simulink model "Hell_ix_System_Architecture"  (R2022b)
settings: Solver=VariableStepAuto  StartTime=0.0  StopTime=10.0  RelTol=1e-3
(part 2 of 2)

== system Hell_ix_System_Architecture/Trials/Test 1: In-Line Obstacle Race ==
  Bus Element In4 : Inport  PortName=End1_hellix
  Bus Element In3 : Inport  Port=2  PortName=End1_droning
  Bus Element In2 : Inport  Port=3  PortName=Start
  Bus Element In1 : Inport  Port=4  PortName=obs
  Bus Element Out1 : Outport  PortName=Points1_hellix
  Bus Element Out2 : Outport  Port=2  PortName=Points1_droning

== system Hell_ix_System_Architecture/Trials/Test 2: Semicircle Obstacle Race ==
  Bus Element In4 : Inport  PortName=End2_hellix
  Bus Element In3 : Inport  Port=2  PortName=End2_droning
  Bus Element In2 : Inport  Port=3  PortName=Start
  Bus Element In1 : Inport  Port=4  PortName=obs
  Bus Element Out1 : Outport  PortName=Points2_hellix
  Bus Element Out2 : Outport  Port=2  PortName=Points2_droning

== system Hell_ix_System_Architecture/Trials/Test 3: Freestyle Test ==
  Bus Element In1 : Inport  PortName=Start
  Bus Element In2 : Inport  Port=2  PortName=End
  Bus Element Out1 : Outport  PortName=Points3_hellix
  Bus Element Out2 : Outport  Port=2  PortName=Points3_droning

== system Hell_ix_System_Architecture/Trials/Winner Determination ==
  Bus Element In2 : Inport  PortName=Points1_droning
  Bus Element In1 : Inport  Port=2  PortName=Points1_hellix
  Bus Element In3 : Inport  Port=3  PortName=Points2_hellix
  Bus Element In4 : Inport  Port=4  PortName=Points2_droning
  Bus Element In6 : Inport  Port=5  PortName=Points3_droning
  Bus Element In5 : Inport  Port=6  PortName=Points3_hellix
  Bus Element Out1 : Outport  PortName=Winner

== system Hell_ix_System_Architecture/Environment/Materials/Chronometer ==
  Bus Element In1 : Inport  PortName=Start
  Bus Element Out1 : Outport  PortName=End

== system Hell_ix_System_Architecture/Environment/Materials/Horn ==
  Bus Element Out1 : Outport  PortName=Start

== system Hell_ix_System_Architecture/Environment/Materials/Obstacles ==
  Bus Element Out1 : Outport  PortName=obs

== system Hell_ix_System_Architecture/Environment/Materials/Recording Cameras ==
  Bus Element In2 : Inport  PortName=End
  Bus Element In1 : Inport  Port=2  PortName=Start

== system Hell_ix_System_Architecture/Environment/People/Audience ==

== system Hell_ix_System_Architecture/Environment/People/Droning Team Members ==
  Bus Element In1 : Inport  PortName=Start2
  Control Manager Droning : Subsystem
      settings: PortSchema="{\"entries\":[{\"content\":{\"headerSize\":26,\"margin\":15,\"minimumSpacing\":25,\"sides\":[{\"content\":{\"connectorIds\":[\"In1\"]},\"type\":\"ConnectorPlacement.EquallySpacedRectSide\",\"uuid\":\"e97e1fd1-9f1b-43cc-bf15-a23fe97b9f57\"},{\"content\":{\"connectorIds\":[\"Out1\"],\"side\":\"RIGHT\"},\"type\":\"ConnectorPlacement.EquallySpacedRectSide\",\"uuid\":\"b384b9c5-fcee-4054-b020-18cc4d409726\"},{\"content\":{\"connectorIds\":[],\"side\":\"TOP\"},\"type\":\"ConnectorPlacement.EquallySpacedRectSide\",\"uuid\":\"0ff74274-cc13-4bc9-ab97-befa0144ddb0\"},{\"content\":{\"connectorIds\":[],\"side\":\"BOTTOM\"},\"type\":\"ConnectorPlacement.EquallySpacedRectSide\",\"uuid\":\"4b238d12-a85d-41d6-ac28-0fdf4a244d85\"}]},\"type\":\"ConnectorPlacement.EquallySpacedConnector\",\"uuid\":\"32a64cae-dc0e-47e5-be72-f6041fa7e3a1\"}],\"packageUris\":[\"http://schema.mathworks.com/mf0/Connector/R2020b\"],\"version\":\"1.0\"}"
  Rest of the Droning Team : Subsystem
      settings: PortSchema="{\"entries\":[{\"content\":{\"headerSize\":26,\"margin\":15,\"minimumSpacing\":25,\"sides\":[{\"content\":{\"connectorIds\":[]},\"type\":\"ConnectorPlacement.EquallySpacedRectSide\",\"uuid\":\"e97e1fd1-9f1b-43cc-bf15-a23fe97b9f57\"},{\"content\":{\"connectorIds\":[],\"side\":\"RIGHT\"},\"type\":\"ConnectorPlacement.EquallySpacedRectSide\",\"uuid\":\"b384b9c5-fcee-4054-b020-18cc4d409726\"},{\"content\":{\"connectorIds\":[],\"side\":\"TOP\"},\"type\":\"ConnectorPlacement.EquallySpacedRectSide\",\"uuid\":\"0ff74274-cc13-4bc9-ab97-befa0144ddb0\"}]},\"type\":\"ConnectorPlacement.EquallySpacedConnector\",\"uuid\":\"32a64cae-dc0e-47e5-be72-f6041fa7e3a1\"}],\"packageUris\":[\"http://schema.mathworks.com/mf0/Connector/R2020b\"],\"version\":\"1.0\"}"
  Bus Element Out1 : Outport  PortName=exec_prog2
  wires:
  Bus Element In1/1 -> Control Manager Droning/1(Start2)
  Control Manager Droning/1(exec_prog2) -> Bus Element Out1/1

== system Hell_ix_System_Architecture/Environment/People/Hell-ix Team Members ==
  Bus Element In1 : Inport  PortName=Start
  Control Manager Hell-ix : Subsystem
      settings: PortSchema="{\"entries\":[{\"content\":{\"headerSize\":26,\"margin\":15,\"minimumSpacing\":25,\"sides\":[{\"content\":{\"connectorIds\":[]},\"type\":\"ConnectorPlacement.EquallySpacedRectSide\",\"uuid\":\"e97e1fd1-9f1b-43cc-bf15-a23fe97b9f57\"},{\"content\":{\"connectorIds\":[\"Out1\"],\"side\":\"RIGHT\"},\"type\":\"ConnectorPlacement.EquallySpacedRectSide\",\"uuid\":\"b384b9c5-fcee-4054-b020-18cc4d409726\"},{\"content\":{\"connectorIds\":[\"Out2\"],\"side\":\"TOP\"},\"type\":\"ConnectorPlacement.EquallySpacedRectSide\",\"uuid\":\"0ff74274-cc13-4bc9-ab97-befa0144ddb0\"},{\"content\":{\"connectorIds\":[\"In1\"],\"side\":\"BOTTOM\"},\"type\":\"ConnectorPlacement.EquallySpacedRectSide\",\"uuid\":\"4b238d12-a85d-41d6-ac28-0fdf4a244d85\"}]},\"type\":\"ConnectorPlacement.EquallySpacedConnector\",\"uuid\":\"32a64cae-dc0e-47e5-be72-f6041fa7e3a1\"}],\"packageUris\":[\"http://schema.mathworks.com/mf0/Connector/R2020b\"],\"version\":\"1.0\"}"
  Rest of the Hell-ix Team : Subsystem
      settings: PortSchema="{\"entries\":[{\"content\":{\"headerSize\":26,\"margin\":15,\"minimumSpacing\":25,\"sides\":[{\"content\":{\"connectorIds\":[]},\"type\":\"ConnectorPlacement.EquallySpacedRectSide\",\"uuid\":\"e97e1fd1-9f1b-43cc-bf15-a23fe97b9f57\"},{\"content\":{\"connectorIds\":[],\"side\":\"RIGHT\"},\"type\":\"ConnectorPlacement.EquallySpacedRectSide\",\"uuid\":\"b384b9c5-fcee-4054-b020-18cc4d409726\"},{\"content\":{\"connectorIds\":[],\"side\":\"TOP\"},\"type\":\"ConnectorPlacement.EquallySpacedRectSide\",\"uuid\":\"0ff74274-cc13-4bc9-ab97-befa0144ddb0\"}]},\"type\":\"ConnectorPlacement.EquallySpacedConnector\",\"uuid\":\"32a64cae-dc0e-47e5-be72-f6041fa7e3a1\"}],\"packageUris\":[\"http://schema.mathworks.com/mf0/Connector/R2020b\"],\"version\":\"1.0\"}"
  Bus Element Out1 : Outport  PortName=exec_prog
  Bus Element Out2 : Outport  Port=2  PortName=config
  wires:
  Control Manager Hell-ix/2(exec_prog) -> Bus Element Out1/1
  Bus Element In1/1 -> Control Manager Hell-ix/1(Start)
  Control Manager Hell-ix/1(config) -> Bus Element Out2/1

== system Hell_ix_System_Architecture/Hell-ix/CrazyFlie 2.1/AI-deck ==
  Bus Element In3 : Inport  PortName=obs
  Bus Element In1 : Inport  Port=2  PortName=MalePins
  Bus Element In2 : Inport  Port=3  PortName=Power
  Camera : Subsystem
      settings: PortSchema="{\"entries\":[{\"content\":{\"headerSize\":26,\"margin\":15,\"minimumSpacing\":25,\"sides\":[{\"content\":{\"connectorIds\":[\"In1\"]},\"type\":\"ConnectorPlacement.EquallySpacedRectSide\",\"uuid\":\"e97e1fd1-9f1b-43cc-bf15-a23fe97b9f57\"},{\"content\":{\"connectorIds\":[\"Out1\"],\"side\":\"RIGHT\"},\"type\":\"ConnectorPlacement.EquallySpacedRectSide\",\"uuid\":\"b384b9c5-fcee-4054-b020-18cc4d409726\"},{\"content\":{\"connectorIds\":[],\"side\":\"TOP\"},\"type\":\"ConnectorPlacement.EquallySpacedRectSide\",\"uuid\":\"0ff74274-cc13-4bc9-ab97-befa0144ddb0\"}]},\"type\":\"ConnectorPlacement.EquallySpacedConnector\",\"uuid\":\"32a64cae-dc0e-47e5-be72-f6041fa7e3a1\"}],\"packageUris\":[\"http://schema.mathworks.com/mf0/Connector/R2020b\"],\"version\":\"1.0\"}"
  GPA8 : Subsystem
      settings: PortSchema="{\"entries\":[{\"content\":{\"headerSize\":26,\"margin\":15,\"minimumSpacing\":25,\"sides\":[{\"content\":{\"connectorIds\":[]},\"type\":\"ConnectorPlacement.EquallySpacedRectSide\",\"uuid\":\"e97e1fd1-9f1b-43cc-bf15-a23fe97b9f57\"},{\"content\":{\"connectorIds\":[],\"side\":\"RIGHT\"},\"type\":\"ConnectorPlacement.EquallySpacedRectSide\",\"uuid\":\"b384b9c5-fcee-4054-b020-18cc4d409726\"},{\"content\":{\"connectorIds\":[],\"side\":\"TOP\"},\"type\":\"ConnectorPlacement.EquallySpacedRectSide\",\"uuid\":\"0ff74274-cc13-4bc9-ab97-befa0144ddb0\"}]},\"type\":\"ConnectorPlacement.EquallySpacedConnector\",\"uuid\":\"32a64cae-dc0e-47e5-be72-f6041fa7e3a1\"}],\"packageUris\":[\"http://schema.mathworks.com/mf0/Connector/R2020b\"],\"version\":\"1.0\"}"
  Bus Element Out1 : Outport  PortName=VideoBus
  wires:
  Camera/1(OutBus) -> Bus Element Out1/1
  Bus Element In3/1 -> Camera/1(obs)

== system Hell_ix_System_Architecture/Hell-ix/CrazyFlie 2.1/Battery ==
  Bus Element In1 : Inport  PortName=hold
  Bus Element Out1 : Outport  PortName=Power

== system Hell_ix_System_Architecture/Hell-ix/CrazyFlie 2.1/Battery Holder Deck ==
  Bus Element In1 : Inport  PortName=MalePins
  Bus Element Out1 : Outport  PortName=hold

== system Hell_ix_System_Architecture/Hell-ix/CrazyFlie 2.1/CCW Helix 1 ==
  Bus Element In1 : Inport  PortName=rotate

== system Hell_ix_System_Architecture/Hell-ix/CrazyFlie 2.1/CCW Helix 2 ==
  Bus Element In1 : Inport  PortName=rotate

== system Hell_ix_System_Architecture/Hell-ix/CrazyFlie 2.1/CW Helix 1 ==
  Bus Element In1 : Inport  PortName=rotate

== system Hell_ix_System_Architecture/Hell-ix/CrazyFlie 2.1/CW Helix 2 ==
  Bus Element In1 : Inport  PortName=rotate

== system Hell_ix_System_Architecture/Hell-ix/CrazyFlie 2.1/Charge Socket ==
  Bus Element Out1 : Outport  PortName=Power

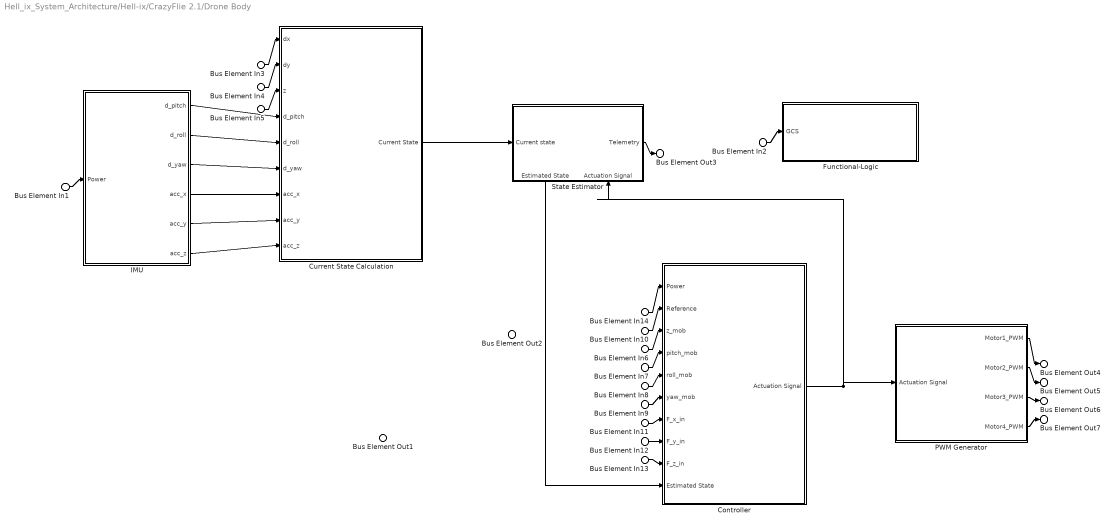
== system Hell_ix_System_Architecture/Hell-ix/CrazyFlie 2.1/Drone Body ==
  Bus Element In11 : Inport  PortName=F_x_in
  Bus Element In12 : Inport  Port=2  PortName=F_y_in
  Bus Element In13 : Inport  Port=3  PortName=F_z_in
  Bus Element In5 : Inport  Port=4  PortName=z
  Bus Element In4 : Inport  Port=5  PortName=dy
  Bus Element In3 : Inport  Port=6  PortName=dx
  Bus Element In2 : Inport  Port=7  PortName=GCS
  Bus Element In1 : Inport  Port=8  PortName=Power
  Bus Element In14 : Inport  Port=8  PortName=Power
  Bus Element In6 : Inport  Port=9  PortName=z_mob
  Bus Element In7 : Inport  Port=10  PortName=pitch_mob
  Bus Element In8 : Inport  Port=11  PortName=roll_mob
  Bus Element In9 : Inport  Port=12  PortName=yaw_mob
  Bus Element In10 : Inport  Port=13  PortName=TelemetryRadio
  Controller : Subsystem
      settings: PortSchema="{\"entries\":[{\"content\":{\"headerSize\":26,\"margin\":15,\"minimumSpacing\":25,\"sides\":[{\"content\":{\"connectorIds\":[\"In1\",\"In6\",\"In2\",\"In3\",\"In4\",\"In5\",\"In7\",\"In8\",\"In9\",\"In10\"]},\"type\":\"ConnectorPlacement.EquallySpacedRectSide\",\"uuid\":\"05353883-9549-4dc8-9a1c-5d1ae12c1484\"},{\"content\":{\"connectorIds\":[\"Out1\"],\"side\":\"RIGHT\"},\"type\":\"ConnectorPlacement.EquallySpacedRectSide\",\"uuid\":\"006c1520-45b5-4971-bef2-ea03737e2b23\"},{\"content\":{\"connectorIds\":[],\"side\":\"TOP\"},\"type\":\"ConnectorPlacement.EquallySpacedRectSide\",\"uuid\":\"e61f6cee-2c78-4df2-8cd1-114268c994e4\"}]},\"type\":\"ConnectorPlacement.EquallySpacedConnector\",\"uuid\":\"e2af53a5-fa78-4528-a754-d30d2cd5caf8\"}],\"packageUris\":[\"http://schema.mathworks.com/mf0/Connector/R2020b\"],\"version\":\"1.0\"}"
  Current State Calculation : Subsystem
      settings: PortSchema="{\"entries\":[{\"content\":{\"headerSize\":26,\"margin\":15,\"minimumSpacing\":25,\"sides\":[{\"content\":{\"connectorIds\":[\"In3\",\"In2\",\"In4\",\"In5\",\"In1\",\"In6\",\"In7\",\"In8\",\"In9\"]},\"type\":\"ConnectorPlacement.EquallySpacedRectSide\",\"uuid\":\"85361f62-a72a-43f7-8205-2bd06b4635eb\"},{\"content\":{\"connectorIds\":[\"Out1\"],\"side\":\"RIGHT\"},\"type\":\"ConnectorPlacement.EquallySpacedRectSide\",\"uuid\":\"785bca03-4c5c-4ff5-9bb5-891ad5972055\"},{\"content\":{\"connectorIds\":[],\"side\":\"TOP\"},\"type\":\"ConnectorPlacement.EquallySpacedRectSide\",\"uuid\":\"4b8cfef5-38ba-456f-a828-b5cb7f165aef\"},{\"content\":{\"connectorIds\":[],\"side\":\"BOTTOM\"},\"type\":\"ConnectorPlacement.EquallySpacedRectSide\",\"uuid\":\"ba702fc0-1fe6-457d-9dcb-728a63d76caf\"}]},\"type\":\"ConnectorPlacement.EquallySpacedConnector\",\"uuid\":\"8dffc657-0173-4421-b98e-59d56a4d09a6\"}],\"packageUris\":[\"http://schema.mathworks.com/mf0/Connector/R2020b\"],\"version\":\"1.0\"}"
  Functional-Logic : Subsystem
      settings: PortSchema="{\"entries\":[{\"content\":{\"headerSize\":26,\"margin\":15,\"minimumSpacing\":25,\"sides\":[{\"content\":{\"connectorIds\":[\"In1\"]},\"type\":\"ConnectorPlacement.EquallySpacedRectSide\",\"uuid\":\"e97e1fd1-9f1b-43cc-bf15-a23fe97b9f57\"},{\"content\":{\"connectorIds\":[],\"side\":\"RIGHT\"},\"type\":\"ConnectorPlacement.EquallySpacedRectSide\",\"uuid\":\"b384b9c5-fcee-4054-b020-18cc4d409726\"},{\"content\":{\"connectorIds\":[],\"side\":\"TOP\"},\"type\":\"ConnectorPlacement.EquallySpacedRectSide\",\"uuid\":\"0ff74274-cc13-4bc9-ab97-befa0144ddb0\"}]},\"type\":\"ConnectorPlacement.EquallySpacedConnector\",\"uuid\":\"32a64cae-dc0e-47e5-be72-f6041fa7e3a1\"}],\"packageUris\":[\"http://schema.mathworks.com/mf0/Connector/R2020b\"],\"version\":\"1.0\"}"
  IMU : Subsystem
      settings: PortSchema="{\"entries\":[{\"content\":{\"headerSize\":26,\"margin\":15,\"minimumSpacing\":25,\"sides\":[{\"content\":{\"connectorIds\":[\"In1\"]},\"type\":\"ConnectorPlacement.EquallySpacedRectSide\",\"uuid\":\"85361f62-a72a-43f7-8205-2bd06b4635eb\"},{\"content\":{\"connectorIds\":[\"Out1\",\"Out2\",\"Out3\",\"Out4\",\"Out5\",\"Out6\"],\"side\":\"RIGHT\"},\"type\":\"ConnectorPlacement.EquallySpacedRectSide\",\"uuid\":\"785bca03-4c5c-4ff5-9bb5-891ad5972055\"},{\"content\":{\"connectorIds\":[],\"side\":\"TOP\"},\"type\":\"ConnectorPlacement.EquallySpacedRectSide\",\"uuid\":\"4b8cfef5-38ba-456f-a828-b5cb7f165aef\"}]},\"type\":\"ConnectorPlacement.EquallySpacedConnector\",\"uuid\":\"8dffc657-0173-4421-b98e-59d56a4d09a6\"}],\"packageUris\":[\"http://schema.mathworks.com/mf0/Connector/R2020b\"],\"version\":\"1.0\"}"
  PWM Generator : Subsystem
      settings: PortSchema="{\"entries\":[{\"content\":{\"headerSize\":26,\"margin\":15,\"minimumSpacing\":25,\"sides\":[{\"content\":{\"connectorIds\":[\"In1\"]},\"type\":\"ConnectorPlacement.EquallySpacedRectSide\",\"uuid\":\"05353883-9549-4dc8-9a1c-5d1ae12c1484\"},{\"content\":{\"connectorIds\":[\"Out1\",\"Out2\",\"Out3\",\"Out4\"],\"side\":\"RIGHT\"},\"type\":\"ConnectorPlacement.EquallySpacedRectSide\",\"uuid\":\"006c1520-45b5-4971-bef2-ea03737e2b23\"},{\"content\":{\"connectorIds\":[],\"side\":\"TOP\"},\"type\":\"ConnectorPlacement.EquallySpacedRectSide\",\"uuid\":\"e61f6cee-2c78-4df2-8cd1-114268c994e4\"}]},\"type\":\"ConnectorPlacement.EquallySpacedConnector\",\"uuid\":\"e2af53a5-fa78-4528-a754-d30d2cd5caf8\"}],\"packageUris\":[\"http://schema.mathworks.com/mf0/Connector/R2020b\"],\"version\":\"1.0\"}"
  State Estimator : Subsystem
      settings: PortSchema="{\"entries\":[{\"content\":{\"headerSize\":26,\"margin\":15,\"minimumSpacing\":25,\"sides\":[{\"content\":{\"connectorIds\":[\"In1\"]},\"type\":\"ConnectorPlacement.EquallySpacedRectSide\",\"uuid\":\"05353883-9549-4dc8-9a1c-5d1ae12c1484\"},{\"content\":{\"connectorIds\":[\"Out1\"],\"side\":\"RIGHT\"},\"type\":\"ConnectorPlacement.EquallySpacedRectSide\",\"uuid\":\"006c1520-45b5-4971-bef2-ea03737e2b23\"},{\"content\":{\"connectorIds\":[],\"side\":\"TOP\"},\"type\":\"ConnectorPlacement.EquallySpacedRectSide\",\"uuid\":\"e61f6cee-2c78-4df2-8cd1-114268c994e4\"},{\"content\":{\"connectorIds\":[\"Out2\",\"In2\"],\"side\":\"BOTTOM\"},\"type\":\"ConnectorPlacement.EquallySpacedRectSide\",\"uuid\":\"d4686ce2-6bf9-4421-adae-f62b00313f34\"}]},\"type\":\"ConnectorPlacement.EquallySpacedConnector\",\"uuid\":\"e2af53a5-fa78-4528-a754-d30d2cd5caf8\"}],\"packageUris\":[\"http://schema.mathworks.com/mf0/Connector/R2020b\"],\"version\":\"1.0\"}"
  Bus Element Out2 : Outport  PortName=MalePins
  Bus Element Out1 : Outport  Port=2  PortName=hold0
  Bus Element Out3 : Outport  Port=3  PortName=Telemetry
  Bus Element Out4 : Outport  Port=4  PortName=Motor1_PWM
  Bus Element Out5 : Outport  Port=5  PortName=Motor2_PWM
  Bus Element Out6 : Outport  Port=6  PortName=Motor3_PWM
  Bus Element Out7 : Outport  Port=7  PortName=Motor4_PWM
  wires:
  IMU/4(acc_x) -> Current State Calculation/7(acc_x)
  IMU/1(d_pitch) -> Current State Calculation/5(d_pitch)
  IMU/5(acc_y) -> Current State Calculation/8(acc_y)
  IMU/2(d_roll) -> Current State Calculation/1(d_roll)
  IMU/6(acc_z) -> Current State Calculation/9(acc_z)
  IMU/3(d_yaw) -> Current State Calculation/6(d_yaw)
  Bus Element In3/1 -> Current State Calculation/3(dx)
  Bus Element In4/1 -> Current State Calculation/2(dy)
  Bus Element In5/1 -> Current State Calculation/4(z)
  State Estimator/1(Telemetry) -> Bus Element Out3/1
  Bus Element In10/1 -> Controller/6(Reference)
  Bus Element In9/1 -> Controller/5(yaw_mob)
  State Estimator/2(Estimated State) -> Controller/10(Estimated State)
  Bus Element In6/1 -> Controller/2(z_mob)
  Bus Element In8/1 -> Controller/4(roll_mob)
  Controller/1(Actuation Signal) -> PWM Generator/1(Actuation Signal), State Estimator/2(Actuation Signal)
  Bus Element In7/1 -> Controller/3(pitch_mob)
  Current State Calculation/1(Current State) -> State Estimator/1(Current state)
  PWM Generator/1(Motor1_PWM) -> Bus Element Out4/1
  PWM Generator/2(Motor2_PWM) -> Bus Element Out5/1
  PWM Generator/3(Motor3_PWM) -> Bus Element Out6/1
  PWM Generator/4(Motor4_PWM) -> Bus Element Out7/1
  Bus Element In11/1 -> Controller/7(F_x_in)
  Bus Element In12/1 -> Controller/8(F_y_in)
  Bus Element In13/1 -> Controller/9(F_z_in)
  Bus Element In2/1 -> Functional-Logic/1(GCS)
  Bus Element In1/1 -> IMU/1(Power)
  Bus Element In14/1 -> Controller/1(Power)

== system Hell_ix_System_Architecture/Hell-ix/CrazyFlie 2.1/Environment Perturbations ==
  Bus Element In1 : Inport  PortName=environment
  Bus Element Out1 : Outport  PortName=F_x_in
  Bus Element Out2 : Outport  Port=2  PortName=F_y_in
  Bus Element Out3 : Outport  Port=3  PortName=F_z_in

== system Hell_ix_System_Architecture/Hell-ix/CrazyFlie 2.1/Flow Deck ==
  Bus Element In1 : Inport  PortName=MalePins
  Bus Element In2 : Inport  Port=2  PortName=Power
  PMW3901 Optical Sensor : Subsystem
      settings: PortSchema="{\"entries\":[{\"content\":{\"headerSize\":26,\"margin\":15,\"minimumSpacing\":25,\"sides\":[{\"content\":{\"connectorIds\":[\"Out1\",\"Out2\"]},\"type\":\"ConnectorPlacement.EquallySpacedRectSide\",\"uuid\":\"e97e1fd1-9f1b-43cc-bf15-a23fe97b9f57\"},{\"content\":{\"connectorIds\":[],\"side\":\"RIGHT\"},\"type\":\"ConnectorPlacement.EquallySpacedRectSide\",\"uuid\":\"b384b9c5-fcee-4054-b020-18cc4d409726\"},{\"content\":{\"connectorIds\":[],\"side\":\"TOP\"},\"type\":\"ConnectorPlacement.EquallySpacedRectSide\",\"uuid\":\"0ff74274-cc13-4bc9-ab97-befa0144ddb0\"}]},\"type\":\"ConnectorPlacement.EquallySpacedConnector\",\"uuid\":\"32a64cae-dc0e-47e5-be72-f6041fa7e3a1\"}],\"packageUris\":[\"http://schema.mathworks.com/mf0/Connector/R2020b\"],\"version\":\"1.0\"}"
  VL53L1x ToF Sensor : Subsystem
      settings: PortSchema="{\"entries\":[{\"content\":{\"headerSize\":26,\"margin\":15,\"minimumSpacing\":25,\"sides\":[{\"content\":{\"connectorIds\":[\"Out1\"]},\"type\":\"ConnectorPlacement.EquallySpacedRectSide\",\"uuid\":\"e97e1fd1-9f1b-43cc-bf15-a23fe97b9f57\"},{\"content\":{\"connectorIds\":[],\"side\":\"RIGHT\"},\"type\":\"ConnectorPlacement.EquallySpacedRectSide\",\"uuid\":\"b384b9c5-fcee-4054-b020-18cc4d409726\"},{\"content\":{\"connectorIds\":[],\"side\":\"TOP\"},\"type\":\"ConnectorPlacement.EquallySpacedRectSide\",\"uuid\":\"0ff74274-cc13-4bc9-ab97-befa0144ddb0\"}]},\"type\":\"ConnectorPlacement.EquallySpacedConnector\",\"uuid\":\"32a64cae-dc0e-47e5-be72-f6041fa7e3a1\"}],\"packageUris\":[\"http://schema.mathworks.com/mf0/Connector/R2020b\"],\"version\":\"1.0\"}"
  Bus Element Out2 : Outport  PortName=dx
  Bus Element Out3 : Outport  Port=2  PortName=dy
  Bus Element Out1 : Outport  Port=3  PortName=z
  wires:
  VL53L1x ToF Sensor/1(z) -> Bus Element Out1/1
  PMW3901 Optical Sensor/1(dx) -> Bus Element Out2/1
  PMW3901 Optical Sensor/2(dy) -> Bus Element Out3/1

== system Hell_ix_System_Architecture/Hell-ix/CrazyFlie 2.1/LED Ring Deck ==
  Bus Element In1 : Inport  PortName=MalePins
  Bus Element In2 : Inport  Port=2  PortName=Power
  Bus Element In3 : Inport  Port=3  PortName=LED_cmds

== system Hell_ix_System_Architecture/Hell-ix/CrazyFlie 2.1/Motor 1 ==
  Bus Element In2 : Inport  PortName=Power
  Bus Element In3 : Inport  Port=2  PortName=Motor1_PWM
  Bus Element In1 : Inport  Port=3  PortName=hold
  Bus Element Out2 : Outport  PortName=rotate

== system Hell_ix_System_Architecture/Hell-ix/CrazyFlie 2.1/Motor 2 ==
  Bus Element In2 : Inport  PortName=Power
  Bus Element In3 : Inport  Port=2  PortName=Motor2_PWM
  Bus Element In1 : Inport  Port=3  PortName=hold
  Bus Element Out2 : Outport  PortName=rotate

== system Hell_ix_System_Architecture/Hell-ix/CrazyFlie 2.1/Motor 3 ==
  Bus Element In2 : Inport  PortName=Power
  Bus Element In3 : Inport  Port=2  PortName=Motor3_PWM
  Bus Element In1 : Inport  Port=3  PortName=hold
  Bus Element Out2 : Outport  PortName=rotate

== system Hell_ix_System_Architecture/Hell-ix/CrazyFlie 2.1/Motor 4 ==
  Bus Element In2 : Inport  PortName=Power
  Bus Element In3 : Inport  Port=2  PortName=Motor4_PWM
  Bus Element In1 : Inport  Port=3  PortName=hold
  Bus Element Out2 : Outport  PortName=rotate

== system Hell_ix_System_Architecture/Hell-ix/CrazyFlie 2.1/Motor Arm 1 ==
  Bus Element In1 : Inport  PortName=hold0
  Bus Element Out1 : Outport  PortName=hold

== system Hell_ix_System_Architecture/Hell-ix/CrazyFlie 2.1/Motor Arm 2 ==
  Bus Element In1 : Inport  PortName=hold0
  Bus Element Out1 : Outport  PortName=hold

== system Hell_ix_System_Architecture/Hell-ix/CrazyFlie 2.1/Motor Arm 3 ==
  Bus Element In1 : Inport  PortName=hold0
  Bus Element Out1 : Outport  PortName=hold

== system Hell_ix_System_Architecture/Hell-ix/CrazyFlie 2.1/Motor Arm 4 ==
  Bus Element In1 : Inport  PortName=hold0
  Bus Element Out1 : Outport  PortName=hold

== system Hell_ix_System_Architecture/Hell-ix/CrazyFlie 2.1/Power Supply Board ==
  Bus Element In2 : Inport  PortName=Power
  Bus Element In1 : Inport  Port=2  PortName=Bat_Power
  Bus Element Out1 : Outport  PortName=5 V

== system Hell_ix_System_Architecture/Hell-ix/Ground Control Station/Commands ==
  Bus Element In1 : Inport  PortName=pos_x_out
  Bus Element In2 : Inport  Port=2  PortName=pos_y_out
  Bus Element In3 : Inport  Port=3  PortName=pos_z_out
  Bus Element In9 : Inport  Port=4  PortName=yaw_out
  Bus Element In5 : Inport  Port=5  PortName=LED_conf
  Bus Element Out2 : Outport  PortName=Telemetry_USB
  Bus Element Out1 : Outport  Port=2  PortName=GCSCmds

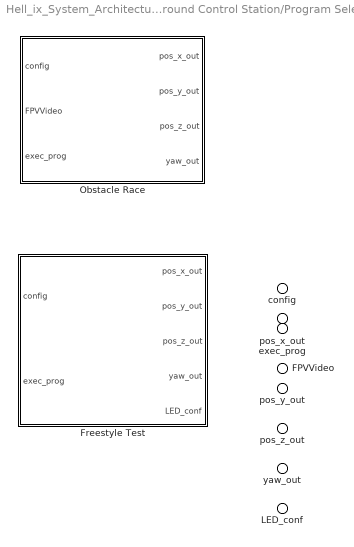
== system Hell_ix_System_Architecture/Hell-ix/Ground Control Station/Program Selection ==
  config : Inport
  exec_prog : Inport  Port=2
  FPVVideo : Inport  Port=3
  Freestyle Test : Subsystem  Variant=on  VariantControlMode=label  VariantControl=Choice  LabelModeActiveChoice=true
      settings: PortSchema="{\"entries\":[{\"content\":{\"headerSize\":38,\"margin\":15,\"minimumSpacing\":25,\"sides\":[{\"content\":{\"connectorIds\":[\"In1\",\"In2\"]},\"type\":\"ConnectorPlacement.EquallySpacedRectSide\",\"uuid\":\"61491797-d554-4a74-923e-4bee7d1a8f93\"},{\"content\":{\"connectorIds\":[\"Out1\",\"Out2\",\"Out3\",\"Out4\",\"Out5\"],\"side\":\"RIGHT\"},\"type\":\"ConnectorPlacement.EquallySpacedRectSide\",\"uuid\":\"68e3b5ad-c508-4145-a439-f07408910c2d\"},{\"content\":{\"connectorIds\":[],\"side\":\"TOP\"},\"type\":\"ConnectorPlacement.EquallySpacedRectSide\",\"uuid\":\"f52cb127-a246-45d5-a620-fd9d5ecf46f3\"}]},\"type\":\"ConnectorPlacement.EquallySpacedConnector\",\"uuid\":\"13f104e8-deb7-48c1-a5c8-cc1a7de63fd1\"}],\"packageUris\":[\"http://schema.mathworks.com/mf0/Connector/R2020b\"],\"version\":\"1.0\"}"
  Obstacle Race : Subsystem  VariantControl=true
      settings: PortSchema="{\"entries\":[{\"content\":{\"headerSize\":26,\"margin\":15,\"minimumSpacing\":25,\"sides\":[{\"content\":{\"connectorIds\":[\"In1\",\"In2\",\"In3\"]},\"type\":\"ConnectorPlacement.EquallySpacedRectSide\",\"uuid\":\"f7f1756e-cfe9-4344-b124-dfbe0f7c04ad\"},{\"content\":{\"connectorIds\":[\"Out1\",\"Out2\",\"Out3\",\"Out4\"],\"side\":\"RIGHT\"},\"type\":\"ConnectorPlacement.EquallySpacedRectSide\",\"uuid\":\"bb7d52d5-2073-42fa-b0cf-3c07249d6568\"},{\"content\":{\"connectorIds\":[],\"side\":\"TOP\"},\"type\":\"ConnectorPlacement.EquallySpacedRectSide\",\"uuid\":\"d64901eb-ea7a-4324-aad3-6455e652f617\"}]},\"type\":\"ConnectorPlacement.EquallySpacedConnector\",\"uuid\":\"ea70cfab-c316-4cb8-aebf-3c722623f4a5\"}],\"packageUris\":[\"http://schema.mathworks.com/mf0/Connector/R2020b\"],\"version\":\"1.0\"}"
  pos_x_out : Outport
  pos_y_out : Outport  Port=2
  pos_z_out : Outport  Port=3
  yaw_out : Outport  Port=4
  LED_conf : Outport  Port=5

== system Hell_ix_System_Architecture/Environment/People/Droning Team Members/Control Manager Droning ==
  Bus Element In2 : Inport  PortName=Start2
  Bus Element Out2 : Outport  PortName=exec_prog2

== system Hell_ix_System_Architecture/Environment/People/Droning Team Members/Rest of the Droning Team ==

== system Hell_ix_System_Architecture/Environment/People/Hell-ix Team Members/Control Manager Hell-ix ==
  Bus Element In1 : Inport  PortName=Start
  Bus Element Out2 : Outport  PortName=config
  Bus Element Out1 : Outport  Port=2  PortName=exec_prog

== system Hell_ix_System_Architecture/Environment/People/Hell-ix Team Members/Rest of the Hell-ix Team ==

== system Hell_ix_System_Architecture/Hell-ix/CrazyFlie 2.1/AI-deck/Camera ==
  Bus Element In1 : Inport  PortName=obs
  Bus Element Out1 : Outport  PortName=OutBus

== system Hell_ix_System_Architecture/Hell-ix/CrazyFlie 2.1/AI-deck/GPA8 ==

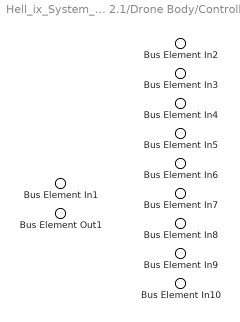
== system Hell_ix_System_Architecture/Hell-ix/CrazyFlie 2.1/Drone Body/Controller ==
  Bus Element In10 : Inport  PortName=Power
  Bus Element In6 : Inport  Port=2  PortName=z_mob
  Bus Element In7 : Inport  Port=3  PortName=pitch_mob
  Bus Element In8 : Inport  Port=4  PortName=roll_mob
  Bus Element In9 : Inport  Port=5  PortName=yaw_mob
  Bus Element In2 : Inport  Port=6  PortName=Reference
  Bus Element In3 : Inport  Port=7  PortName=F_x_in
  Bus Element In4 : Inport  Port=8  PortName=F_y_in
  Bus Element In5 : Inport  Port=9  PortName=F_z_in
  Bus Element In1 : Inport  Port=10  PortName=Estimated State
  Bus Element Out1 : Outport  PortName=Actuation Signal

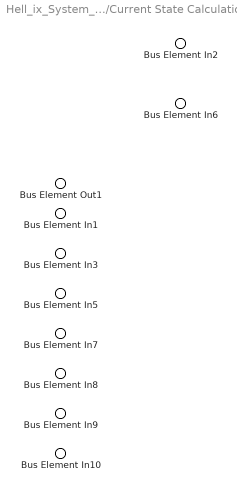
== system Hell_ix_System_Architecture/Hell-ix/CrazyFlie 2.1/Drone Body/Current State Calculation ==
  Bus Element In6 : Inport  PortName=d_roll
  Bus Element In2 : Inport  Port=2  PortName=dy
  Bus Element In1 : Inport  Port=3  PortName=dx
  Bus Element In3 : Inport  Port=4  PortName=z
  Bus Element In5 : Inport  Port=5  PortName=d_pitch
  Bus Element In7 : Inport  Port=6  PortName=d_yaw
  Bus Element In8 : Inport  Port=7  PortName=acc_x
  Bus Element In9 : Inport  Port=8  PortName=acc_y
  Bus Element In10 : Inport  Port=9  PortName=acc_z
  Bus Element Out1 : Outport  PortName=Current State

== system Hell_ix_System_Architecture/Hell-ix/CrazyFlie 2.1/Drone Body/Functional-Logic ==
  Bus Element In1 : Inport  PortName=GCS

== system Hell_ix_System_Architecture/Hell-ix/CrazyFlie 2.1/Drone Body/IMU ==
  Bus Element In1 : Inport  PortName=Power
  Bus Element Out5 : Outport  PortName=d_pitch
  Bus Element Out6 : Outport  Port=2  PortName=d_roll
  Bus Element Out4 : Outport  Port=3  PortName=d_yaw
  Bus Element Out1 : Outport  Port=4  PortName=acc_x
  Bus Element Out2 : Outport  Port=5  PortName=acc_y
  Bus Element Out3 : Outport  Port=6  PortName=acc_z

== system Hell_ix_System_Architecture/Hell-ix/CrazyFlie 2.1/Drone Body/PWM Generator ==
  Bus Element In1 : Inport  PortName=Actuation Signal
  Bus Element Out1 : Outport  PortName=Motor1_PWM
  Bus Element Out2 : Outport  Port=2  PortName=Motor2_PWM
  Bus Element Out3 : Outport  Port=3  PortName=Motor3_PWM
  Bus Element Out4 : Outport  Port=4  PortName=Motor4_PWM

== system Hell_ix_System_Architecture/Hell-ix/CrazyFlie 2.1/Drone Body/State Estimator ==
  Bus Element In1 : Inport  PortName=Current state
  Bus Element In2 : Inport  Port=2  PortName=Actuation Signal
  Bus Element Out2 : Outport  PortName=Telemetry
  Bus Element Out1 : Outport  Port=2  PortName=Estimated State

== system Hell_ix_System_Architecture/Hell-ix/CrazyFlie 2.1/Flow Deck/PMW3901 Optical Sensor ==
  Bus Element Out1 : Outport  PortName=dx
  Bus Element Out2 : Outport  Port=2  PortName=dy

== system Hell_ix_System_Architecture/Hell-ix/CrazyFlie 2.1/Flow Deck/VL53L1x ToF Sensor ==
  Bus Element Out1 : Outport  PortName=z

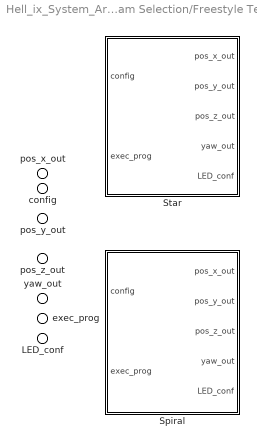
== system Hell_ix_System_Architecture/Hell-ix/Ground Control Station/Program Selection/Freestyle Test ==
  config : Inport
  exec_prog : Inport  Port=2
  Spiral : Subsystem  VariantControl=Choice
      settings: PortSchema="{\"entries\":[{\"content\":{\"headerSize\":26,\"margin\":15,\"minimumSpacing\":25,\"sides\":[{\"content\":{\"connectorIds\":[\"In1\",\"In2\"]},\"type\":\"ConnectorPlacement.EquallySpacedRectSide\",\"uuid\":\"e97e1fd1-9f1b-43cc-bf15-a23fe97b9f57\"},{\"content\":{\"connectorIds\":[\"Out1\",\"Out2\",\"Out3\",\"Out4\",\"Out5\"],\"side\":\"RIGHT\"},\"type\":\"ConnectorPlacement.EquallySpacedRectSide\",\"uuid\":\"b384b9c5-fcee-4054-b020-18cc4d409726\"},{\"content\":{\"connectorIds\":[],\"side\":\"TOP\"},\"type\":\"ConnectorPlacement.EquallySpacedRectSide\",\"uuid\":\"0ff74274-cc13-4bc9-ab97-befa0144ddb0\"}]},\"type\":\"ConnectorPlacement.EquallySpacedConnector\",\"uuid\":\"32a64cae-dc0e-47e5-be72-f6041fa7e3a1\"}],\"packageUris\":[\"http://schema.mathworks.com/mf0/Connector/R2020b\"],\"version\":\"1.0\"}"
  Star : Subsystem  VariantControl=true
      settings: PortSchema="{\"entries\":[{\"content\":{\"headerSize\":26,\"margin\":15,\"minimumSpacing\":25,\"sides\":[{\"content\":{\"connectorIds\":[\"In1\",\"In2\"]},\"type\":\"ConnectorPlacement.EquallySpacedRectSide\",\"uuid\":\"f7f1756e-cfe9-4344-b124-dfbe0f7c04ad\"},{\"content\":{\"connectorIds\":[\"Out2\",\"Out3\",\"Out4\",\"Out5\",\"Out1\"],\"side\":\"RIGHT\"},\"type\":\"ConnectorPlacement.EquallySpacedRectSide\",\"uuid\":\"bb7d52d5-2073-42fa-b0cf-3c07249d6568\"},{\"content\":{\"connectorIds\":[],\"side\":\"TOP\"},\"type\":\"ConnectorPlacement.EquallySpacedRectSide\",\"uuid\":\"d64901eb-ea7a-4324-aad3-6455e652f617\"},{\"content\":{\"connectorIds\":[],\"side\":\"BOTTOM\"},\"type\":\"ConnectorPlacement.EquallySpacedRectSide\",\"uuid\":\"27f2a8cc-c73c-440a-a894-813b156fee90\"}]},\"type\":\"ConnectorPlacement.EquallySpacedConnector\",\"uuid\":\"ea70cfab-c316-4cb8-aebf-3c722623f4a5\"}],\"packageUris\":[\"http://schema.mathworks.com/mf0/Connector/R2020b\"],\"version\":\"1.0\"}"
  pos_x_out : Outport
  pos_y_out : Outport  Port=2
  pos_z_out : Outport  Port=3
  yaw_out : Outport  Port=4
  LED_conf : Outport  Port=5

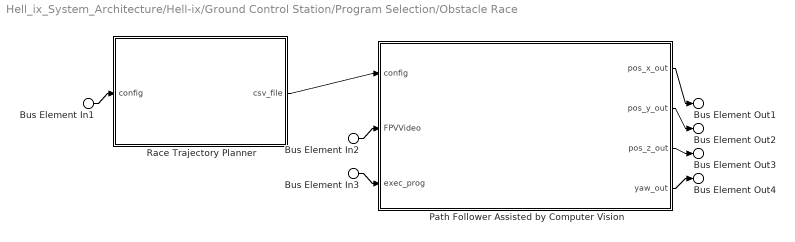
== system Hell_ix_System_Architecture/Hell-ix/Ground Control Station/Program Selection/Obstacle Race ==
  Bus Element In1 : Inport  PortName=config
  Bus Element In2 : Inport  Port=2  PortName=FPVVideo
  Bus Element In3 : Inport  Port=3  PortName=exec_prog
  Path Follower Assisted by Computer Vision : Subsystem
      settings: PortSchema="{\"entries\":[{\"content\":{\"headerSize\":26,\"margin\":15,\"minimumSpacing\":25,\"sides\":[{\"content\":{\"connectorIds\":[\"In1\",\"In2\",\"In3\"]},\"type\":\"ConnectorPlacement.EquallySpacedRectSide\",\"uuid\":\"e97e1fd1-9f1b-43cc-bf15-a23fe97b9f57\"},{\"content\":{\"connectorIds\":[\"Out1\",\"Out2\",\"Out3\",\"Out4\"],\"side\":\"RIGHT\"},\"type\":\"ConnectorPlacement.EquallySpacedRectSide\",\"uuid\":\"b384b9c5-fcee-4054-b020-18cc4d409726\"},{\"content\":{\"connectorIds\":[],\"side\":\"TOP\"},\"type\":\"ConnectorPlacement.EquallySpacedRectSide\",\"uuid\":\"0ff74274-cc13-4bc9-ab97-befa0144ddb0\"}]},\"type\":\"ConnectorPlacement.EquallySpacedConnector\",\"uuid\":\"32a64cae-dc0e-47e5-be72-f6041fa7e3a1\"}],\"packageUris\":[\"http://schema.mathworks.com/mf0/Connector/R2020b\"],\"version\":\"1.0\"}"
  Race Trajectory Planner : Subsystem
      settings: PortSchema="{\"entries\":[{\"content\":{\"headerSize\":26,\"margin\":15,\"minimumSpacing\":25,\"sides\":[{\"content\":{\"connectorIds\":[\"In1\"]},\"type\":\"ConnectorPlacement.EquallySpacedRectSide\",\"uuid\":\"e97e1fd1-9f1b-43cc-bf15-a23fe97b9f57\"},{\"content\":{\"connectorIds\":[\"Out1\"],\"side\":\"RIGHT\"},\"type\":\"ConnectorPlacement.EquallySpacedRectSide\",\"uuid\":\"b384b9c5-fcee-4054-b020-18cc4d409726\"},{\"content\":{\"connectorIds\":[],\"side\":\"TOP\"},\"type\":\"ConnectorPlacement.EquallySpacedRectSide\",\"uuid\":\"0ff74274-cc13-4bc9-ab97-befa0144ddb0\"}]},\"type\":\"ConnectorPlacement.EquallySpacedConnector\",\"uuid\":\"32a64cae-dc0e-47e5-be72-f6041fa7e3a1\"}],\"packageUris\":[\"http://schema.mathworks.com/mf0/Connector/R2020b\"],\"version\":\"1.0\"}"
  Bus Element Out1 : Outport  PortName=pos_x_out
  Bus Element Out2 : Outport  Port=2  PortName=pos_y_out
  Bus Element Out3 : Outport  Port=3  PortName=pos_z_out
  Bus Element Out4 : Outport  Port=4  PortName=yaw_out
  wires:
  Bus Element In1/1 -> Race Trajectory Planner/1(config)
  Race Trajectory Planner/1(csv_file) -> Path Follower Assisted by Computer Vision/1(config)
  Bus Element In2/1 -> Path Follower Assisted by Computer Vision/2(FPVVideo)
  Bus Element In3/1 -> Path Follower Assisted by Computer Vision/3(exec_prog)
  Path Follower Assisted by Computer Vision/1(pos_x_out) -> Bus Element Out1/1
  Path Follower Assisted by Computer Vision/2(pos_y_out) -> Bus Element Out2/1
  Path Follower Assisted by Computer Vision/3(pos_z_out) -> Bus Element Out3/1
  Path Follower Assisted by Computer Vision/4(yaw_out) -> Bus Element Out4/1

== system Hell_ix_System_Architecture/Hell-ix/Ground Control Station/Program Selection/Freestyle Test/Spiral ==
  Bus Element In1 : Inport  PortName=config
  Bus Element In2 : Inport  Port=2  PortName=exec_prog
  Bus Element Out1 : Outport  PortName=pos_x_out
  Bus Element Out2 : Outport  Port=2  PortName=pos_y_out
  Bus Element Out3 : Outport  Port=3  PortName=pos_z_out
  Bus Element Out4 : Outport  Port=4  PortName=yaw_out
  Bus Element Out5 : Outport  Port=5  PortName=LED_conf

== system Hell_ix_System_Architecture/Hell-ix/Ground Control Station/Program Selection/Freestyle Test/Star ==
  Bus Element In1 : Inport  PortName=config
  Bus Element In2 : Inport  Port=2  PortName=exec_prog
  Bus Element Out5 : Outport  PortName=LED_conf
  Bus Element Out1 : Outport  Port=2  PortName=pos_x_out
  Bus Element Out2 : Outport  Port=3  PortName=pos_y_out
  Bus Element Out3 : Outport  Port=4  PortName=pos_z_out
  Bus Element Out4 : Outport  Port=5  PortName=yaw_out

== system Hell_ix_System_Architecture/Hell-ix/Ground Control Station/Program Selection/Obstacle Race/Path Follower Assisted by Computer Vision ==
  Bus Element In1 : Inport  PortName=config
  Bus Element In2 : Inport  Port=2  PortName=FPVVideo
  Bus Element In3 : Inport  Port=3  PortName=exec_prog
  Bus Element Out1 : Outport  PortName=pos_x_out
  Bus Element Out2 : Outport  Port=2  PortName=pos_y_out
  Bus Element Out3 : Outport  Port=3  PortName=pos_z_out
  Bus Element Out4 : Outport  Port=4  PortName=yaw_out

== system Hell_ix_System_Architecture/Hell-ix/Ground Control Station/Program Selection/Obstacle Race/Race Trajectory Planner ==
  Bus Element In1 : Inport  PortName=config
  Bus Element Out1 : Outport  PortName=csv_file
